simulink model "ex4"  (R2020a)
settings: Solver=VariableStepDiscrete  StartTime=0.0  StopTime=10.0  MaxStep=0.01  RelTol=1e-3
settings Model: Creator=반달  LastModifiedBy=반달

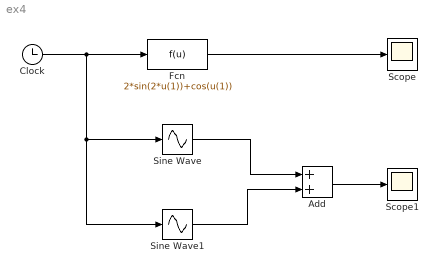
== system ex4 ==
  Add : Sum
  Clock : Clock
  Fcn : Fcn  Expr=2*sin(2*u(1))+cos(u(1))
  Scope : Scope
  Scope1 : Scope
  Sine Wave : Sin  TimeSource=Use external signal  Amplitude=2  Frequency=2  SampleTime=0
  Sine Wave1 : Sin  TimeSource=Use external signal  Phase=pi/2  SampleTime=0
  wires:
  Clock/1 -> Sine Wave1/1, Sine Wave/1, Fcn/1
  Sine Wave/1 -> Add/1
  Sine Wave1/1 -> Add/2
  Add/1 -> Scope1/1
  Fcn/1 -> Scope/1
